simulink library "UltraStick120_Aero_Lib"  (Simulink 8.0)
settings: Solver=ode45  StartTime=0.0  StopTime=10.0  RelTol=1e-3
values from neighbouring files (symbols this model uses):
  AC = miniMUTT_config    [UAV_config.m]    (also in UAV_modelconfig.mat = )
libraries: simulink x2
settings Model: Creator=austinmurch  LastModifiedBy=brtaylor

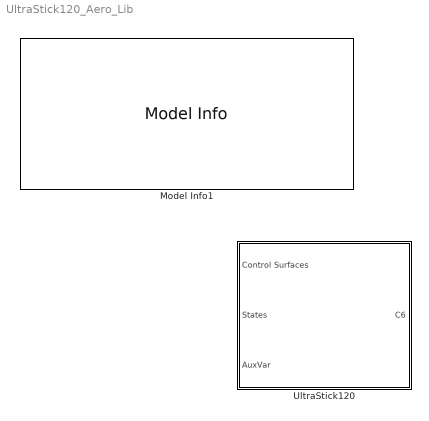
== system UltraStick120_Aero_Lib ==
  Model Info1 : simulink/Model-Wide Utilities/Model Info  InitialBlockCM=None  BlockCM=None  Frame=on  DisplayStringWithTags=|  HorizontalTextAlignment=Left  LeftAlignmentValue=0.02  SourceBlockDiagram=UltraStick120_Aero_Lib  TagMaxNumber=20
      | MODEL INFORMATION
      | FASER Aerodynamic Model Library
      | 
      | University of Minnesota
      | Aerospace Engineering and Mechanics
      | Copyright 2011 Regents of the University of Minnesota. All rights reserved.
      | 
      | == SVN Info ==
      | Last modified by %<LastModifiedBy> on %<LastModificationDate>
  UltraStick120 : Subsystem

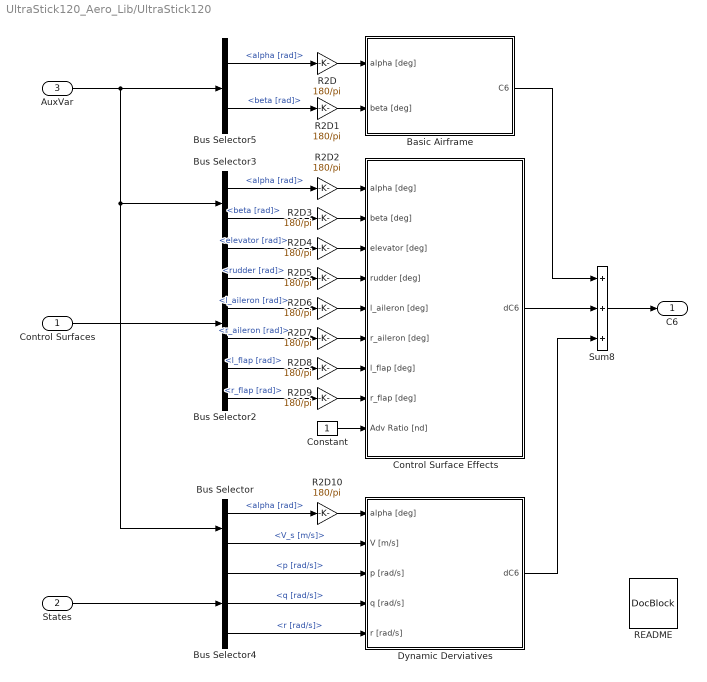
== system UltraStick120_Aero_Lib/UltraStick120 ==
  Control Surfaces : Inport
  States : Inport  Port=2
  AuxVar : Inport  Port=3
  Basic Airframe : Subsystem
  Bus Selector : BusSelector  OutputSignals=WindAxesParam.alpha [rad],WindAxesParam.V_s [m/s]
  Bus Selector2 : BusSelector  OutputSignals=elevator [rad],rudder [rad],l_aileron [rad],r_aileron [rad],l_flap [rad],r_flap [rad]
  Bus Selector3 : BusSelector  OutputSignals=WindAxesParam.alpha [rad],WindAxesParam.beta [rad]
  Bus Selector4 : BusSelector  OutputSignals=AngVel [rad/s].p [rad/s],AngVel [rad/s].q [rad/s],AngVel [rad/s].r [rad/s]
  Bus Selector5 : BusSelector  OutputSignals=WindAxesParam.alpha [rad],WindAxesParam.beta [rad]
  Constant : Constant
  Control Surface Effects : Subsystem
  Dynamic Derviatives : Subsystem
  R2D{,1..10} (11 alike) : Gain  Gain=180/pi
  README : simulink/Model-Wide Utilities/DocBlock  DocumentType=Text
  Sum8 : Sum  Inputs=+++  SaturateOnIntegerOverflow=on  InputSameDT=on  OutDataTypeStr=Inherit: Same as first input
  C6 : Outport
  wires:
  R2D10/1 -> Dynamic Derviatives/1(alpha [deg])
  Bus Selector4/3 -> Dynamic Derviatives/5(r [rad/s])  "<r [rad/s]>"
  Bus Selector4/2 -> Dynamic Derviatives/4(q [rad/s])  "<q [rad/s]>"
  Bus Selector4/1 -> Dynamic Derviatives/3(p [rad/s])  "<p [rad/s]>"
  Bus Selector3/2 -> R2D3/1  "<beta [rad]>"
  Bus Selector3/1 -> R2D2/1  "<alpha [rad]>"
  Bus Selector2/1 -> R2D4/1  "<elevator [rad]>"
  Control Surfaces/1 -> Bus Selector2/1
  Constant/1 -> Control Surface Effects/9(Adv Ratio [nd])
  Basic Airframe/1(C6) -> Sum8/1
  Control Surface Effects/1(dC6) -> Sum8/2
  Dynamic Derviatives/1(dC6) -> Sum8/3
  Sum8/1 -> C6/1
  R2D/1 -> Basic Airframe/1(alpha [deg])
  R2D1/1 -> Basic Airframe/2(beta [deg])
  R2D2/1 -> Control Surface Effects/1(alpha [deg])
  R2D3/1 -> Control Surface Effects/2(beta [deg])
  R2D4/1 -> Control Surface Effects/3(elevator [deg])
  Bus Selector2/2 -> R2D5/1  "<rudder [rad]>"
  R2D5/1 -> Control Surface Effects/4(rudder [deg])
  Bus Selector2/3 -> R2D6/1  "<l_aileron [rad]>"
  Bus Selector2/4 -> R2D7/1  "<r_aileron [rad]>"
  Bus Selector2/5 -> R2D8/1  "<l_flap [rad]>"
  Bus Selector2/6 -> R2D9/1  "<r_flap [rad]>"
  R2D6/1 -> Control Surface Effects/5(l_aileron [deg])
  R2D7/1 -> Control Surface Effects/6(r_aileron [deg])
  R2D8/1 -> Control Surface Effects/7(l_flap [deg])
  R2D9/1 -> Control Surface Effects/8(r_flap [deg])
  Bus Selector5/2 -> R2D1/1  "<beta [rad]>"
  Bus Selector5/1 -> R2D/1  "<alpha [rad]>"
  AuxVar/1 -> Bus Selector/1, Bus Selector3/1, Bus Selector5/1
  Bus Selector/1 -> R2D10/1  "<alpha [rad]>"
  Bus Selector/2 -> Dynamic Derviatives/2(V [m/s])  "<V_s [m/s]>"
  States/1 -> Bus Selector4/1

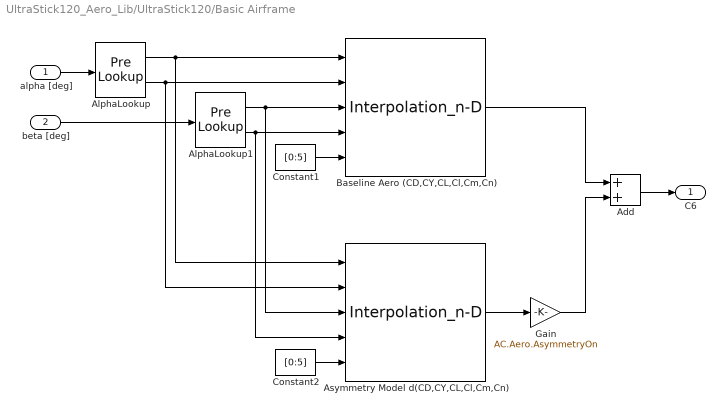
== system UltraStick120_Aero_Lib/UltraStick120/Basic Airframe ==
  alpha [deg] : Inport
  beta [deg] : Inport  Port=2
  Add : Sum
  AlphaLookup : PreLookup  BreakpointsData=AC.Aero.C6_bas.alpha  IndexSearchMethod=Linear search  BeginIndexSearchUsingPreviousIndexResult=on  ExtrapMethod=Linear
  AlphaLookup1 : PreLookup  BreakpointsData=AC.Aero.C6_bas.beta  IndexSearchMethod=Linear search  BeginIndexSearchUsingPreviousIndexResult=on  ExtrapMethod=Linear
  Asymmetry Model d(CD,CY,CL,Cl,Cm,Cn) : Interpolation_n-D  NumberOfTableDimensions=3  Table=AC.Aero.dC6_asym.data  NumSelectionDims=1
      settings: InputPortMap=u0,u1,u2,u3,u4
  Baseline Aero (CD,CY,CL,Cl,Cm,Cn) : Interpolation_n-D  NumberOfTableDimensions=3  Table=AC.Aero.C6_bas.data  NumSelectionDims=1
      settings: InputPortMap=u0,u1,u2,u3,u4
  Constant1 : Constant  Value=[0:5]  OutDataTypeStr=uint32
  Constant2 : Constant  Value=[0:5]  OutDataTypeStr=uint32
  Gain : Gain  Gain=AC.Aero.AsymmetryOn
  C6 : Outport
  wires:
  alpha [deg]/1 -> AlphaLookup/1
  beta [deg]/1 -> AlphaLookup1/1
  AlphaLookup/1 -> Baseline Aero (CD,CY,CL,Cl,Cm,Cn)/1, Asymmetry Model d(CD,CY,CL,Cl,Cm,Cn)/1
  AlphaLookup/2 -> Baseline Aero (CD,CY,CL,Cl,Cm,Cn)/2, Asymmetry Model d(CD,CY,CL,Cl,Cm,Cn)/2
  AlphaLookup1/1 -> Baseline Aero (CD,CY,CL,Cl,Cm,Cn)/3, Asymmetry Model d(CD,CY,CL,Cl,Cm,Cn)/3
  AlphaLookup1/2 -> Baseline Aero (CD,CY,CL,Cl,Cm,Cn)/4, Asymmetry Model d(CD,CY,CL,Cl,Cm,Cn)/4
  Constant1/1 -> Baseline Aero (CD,CY,CL,Cl,Cm,Cn)/5
  Constant2/1 -> Asymmetry Model d(CD,CY,CL,Cl,Cm,Cn)/5
  Baseline Aero (CD,CY,CL,Cl,Cm,Cn)/1 -> Add/1
  Asymmetry Model d(CD,CY,CL,Cl,Cm,Cn)/1 -> Gain/1
  Add/1 -> C6/1
  Gain/1 -> Add/2

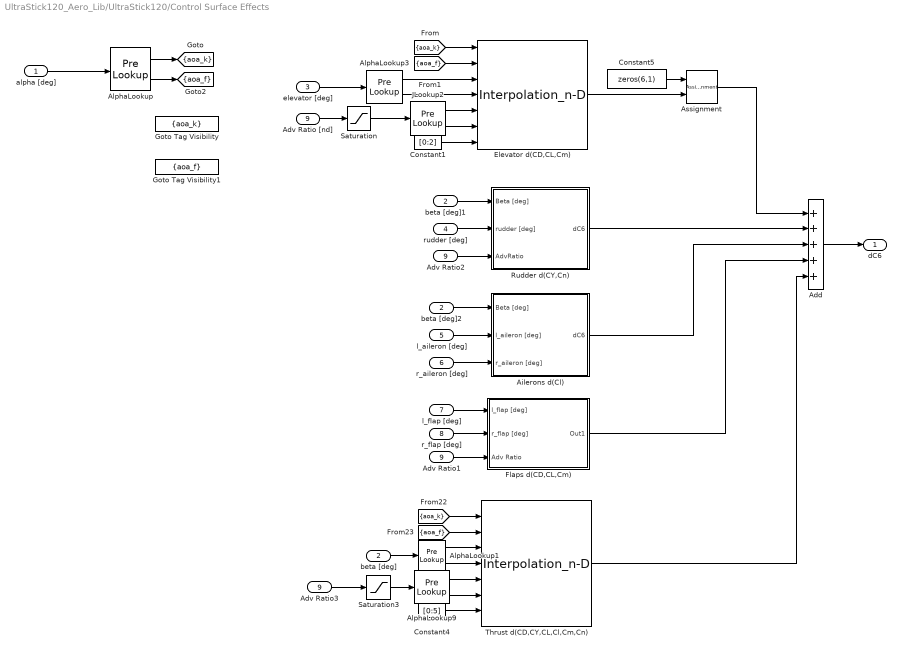
== system UltraStick120_Aero_Lib/UltraStick120/Control Surface Effects ==
  alpha [deg] : Inport
  beta [deg] : Inport  Port=2  PortDimensions=1
  elevator [deg] : Inport  Port=3  PortDimensions=1
  rudder [deg] : Inport  Port=4  PortDimensions=1
  l_aileron [deg] : Inport  Port=5  PortDimensions=1
  r_aileron [deg] : Inport  Port=6  PortDimensions=1
  l_flap [deg] : Inport  Port=7  PortDimensions=1
  r_flap [deg] : Inport  Port=8  PortDimensions=1
  Adv Ratio [nd] : Inport  Port=9
  Add : Sum  Inputs=+++++
  Adv Ratio1 : InportShadow  Port=9
  Adv Ratio2 : InportShadow  Port=9
  Adv Ratio3 : InportShadow  Port=9
  Ailerons d(Cl) : Subsystem
  AlphaLookup : PreLookup  BreakpointsData=AC.Aero.C6_bas.alpha  IndexSearchMethod=Linear search  BeginIndexSearchUsingPreviousIndexResult=on  ExtrapMethod=Linear  UseLastBreakpoint=on
  AlphaLookup1 : PreLookup  BreakpointsData=AC.Aero.C6_bas.beta  IndexSearchMethod=Linear search  BeginIndexSearchUsingPreviousIndexResult=on  ExtrapMethod=Linear  UseLastBreakpoint=on
  AlphaLookup3 : PreLookup  BreakpointsData=AC.Aero.dC3_ele.ele  IndexSearchMethod=Linear search  BeginIndexSearchUsingPreviousIndexResult=on  ExtrapMethod=Linear  UseLastBreakpoint=on
  AlphaLookup9 : PreLookup  BreakpointsData=AC.Aero.dC6_pow.J  IndexSearchMethod=Linear search  BeginIndexSearchUsingPreviousIndexResult=on  ExtrapMethod=Linear  UseLastBreakpoint=on
  Assignment : Assignment  IndexOptions=Index vector (dialog)  Indices=[1 3 5]  OutputSizes=[1 1]
  Constant1 : Constant  Value=[0:2]  OutDataTypeStr=uint32
  Constant4 : Constant  Value=[0:5]  OutDataTypeStr=uint32
  Constant5 : Constant  Value=zeros(6,1)
  Elevator d(CD,CL,Cm) : Interpolation_n-D  NumberOfTableDimensions=4  Table=AC.Aero.dC3_ele.data  NumSelectionDims=1
      settings: InputPortMap=u0,u1,u2,u3,u4,u5,u6
  Flaps d(CD,CL,Cm) : Subsystem
  Goto Tag Visibility : GotoTagVisibility  GotoTag=aoa_k
  Goto Tag Visibility1 : GotoTagVisibility  GotoTag=aoa_f
  JLookup2 : PreLookup  BreakpointsData=AC.Aero.dC3_ele.J  IndexSearchMethod=Linear search  BeginIndexSearchUsingPreviousIndexResult=on  ExtrapMethod=Linear  UseLastBreakpoint=on
  Rudder d(CY,Cn) : Subsystem
  Saturation : Saturate  UpperLimit=max(AC.Aero.dC3_ele.J)  LowerLimit=min(AC.Aero.dC3_ele.J)
  Saturation3 : Saturate  UpperLimit=max(AC.Aero.dC6_pow.J)+eps  LowerLimit=min(AC.Aero.dC6_pow.J)+eps
  Thrust d(CD,CY,CL,Cl,Cm,Cn) : Interpolation_n-D  NumberOfTableDimensions=4  Table=AC.Aero.dC6_pow.data  NumSelectionDims=1
      settings: InputPortMap=u0,u1,u2,u3,u4,u5,u6
  beta [deg]1 : InportShadow  Port=2  PortDimensions=1
  beta [deg]2 : InportShadow  Port=2  PortDimensions=1
  dC6 : Outport  PortDimensions=6
  tag scope: aoa_f=scoped, aoa_k=scoped
  wires:
  alpha [deg]/1 -> AlphaLookup/1
  beta [deg]/1 -> AlphaLookup1/1
  AlphaLookup/1 -> [aoa_k]
  AlphaLookup/2 -> [aoa_f]
  Constant1/1 -> Elevator d(CD,CL,Cm)/7
  [aoa_k] -> Elevator d(CD,CL,Cm)/1
  [aoa_f] -> Elevator d(CD,CL,Cm)/2
  elevator [deg]/1 -> AlphaLookup3/1
  AlphaLookup3/1 -> Elevator d(CD,CL,Cm)/3
  AlphaLookup3/2 -> Elevator d(CD,CL,Cm)/4
  [aoa_k] -> Thrust d(CD,CY,CL,Cl,Cm,Cn)/1
  [aoa_f] -> Thrust d(CD,CY,CL,Cl,Cm,Cn)/2
  AlphaLookup1/1 -> Thrust d(CD,CY,CL,Cl,Cm,Cn)/3
  AlphaLookup1/2 -> Thrust d(CD,CY,CL,Cl,Cm,Cn)/4
  Constant4/1 -> Thrust d(CD,CY,CL,Cl,Cm,Cn)/7
  Elevator d(CD,CL,Cm)/1 -> Assignment/2
  Constant5/1 -> Assignment/1
  Assignment/1 -> Add/1
  Add/1 -> dC6/1
  JLookup2/1 -> Elevator d(CD,CL,Cm)/5
  JLookup2/2 -> Elevator d(CD,CL,Cm)/6
  AlphaLookup9/1 -> Thrust d(CD,CY,CL,Cl,Cm,Cn)/5
  AlphaLookup9/2 -> Thrust d(CD,CY,CL,Cl,Cm,Cn)/6
  Adv Ratio3/1 -> Saturation3/1
  Adv Ratio [nd]/1 -> Saturation/1
  Saturation/1 -> JLookup2/1
  Saturation3/1 -> AlphaLookup9/1
  beta [deg]1/1 -> Rudder d(CY,Cn)/1(Beta [deg])
  rudder [deg]/1 -> Rudder d(CY,Cn)/2(rudder [deg])
  Adv Ratio2/1 -> Rudder d(CY,Cn)/3(AdvRatio)
  r_aileron [deg]/1 -> Ailerons d(Cl)/3(r_aileron [deg])
  l_aileron [deg]/1 -> Ailerons d(Cl)/2(l_aileron [deg])
  beta [deg]2/1 -> Ailerons d(Cl)/1(Beta [deg])
  Adv Ratio1/1 -> Flaps d(CD,CL,Cm)/3(Adv Ratio)
  r_flap [deg]/1 -> Flaps d(CD,CL,Cm)/2(r_flap [deg])
  l_flap [deg]/1 -> Flaps d(CD,CL,Cm)/1(l_flap [deg])
  Rudder d(CY,Cn)/1(dC6) -> Add/2
  Ailerons d(Cl)/1(dC6) -> Add/3
  Flaps d(CD,CL,Cm)/1(Out1) -> Add/4
  Thrust d(CD,CY,CL,Cl,Cm,Cn)/1 -> Add/5

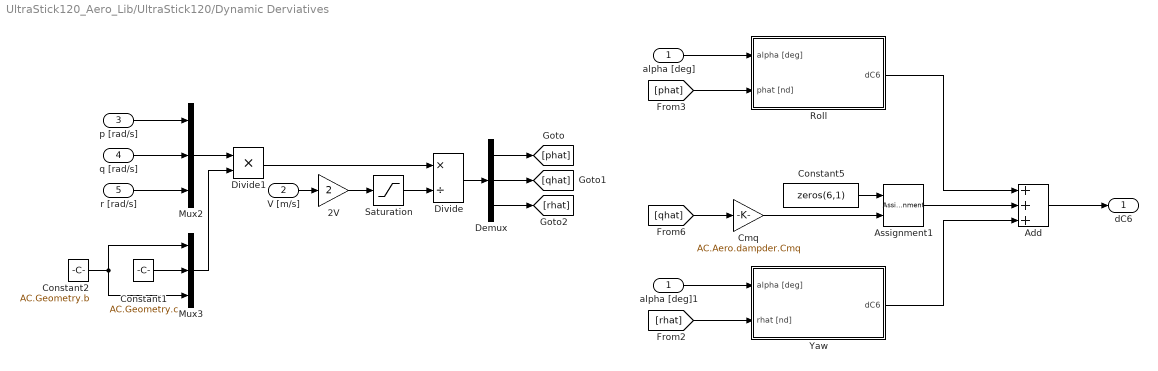
== system UltraStick120_Aero_Lib/UltraStick120/Dynamic Derviatives ==
  alpha [deg] : Inport
  V [m/s] : Inport  Port=2
  p [rad/s] : Inport  Port=3
  q [rad/s] : Inport  Port=4
  r [rad/s] : Inport  Port=5
  2V : Gain  Gain=2
  Add : Sum  Inputs=+++
  Assignment1 : Assignment  IndexOptions=Index vector (dialog)  Indices=5  OutputSizes=[1 1]
  Cmq : Gain  Gain=AC.Aero.dampder.Cmq
  Constant1 : Constant  Value=AC.Geometry.c
  Constant2 : Constant  Value=AC.Geometry.b
  Constant5 : Constant  Value=zeros(6,1)
  Demux : Demux  Outputs=3
  Divide : Product  Inputs=*/
  Divide1 : Product  Inputs=**
  Mux2 : Mux  Inputs=3
  Mux3 : Mux  Inputs=3
  Roll : Subsystem
  Saturation : Saturate  UpperLimit=Inf  LowerLimit=0.001
  Yaw : Subsystem
  alpha [deg]1 : InportShadow
  dC6 : Outport
  wires:
  Yaw/1(dC6) -> Add/3
  Assignment1/1 -> Add/2
  Roll/1(dC6) -> Add/1
  alpha [deg]1/1 -> Yaw/1(alpha [deg])
  alpha [deg]/1 -> Roll/1(alpha [deg])
  Constant5/1 -> Assignment1/1
  [rhat] -> Yaw/2(rhat [nd])
  [phat] -> Roll/2(phat [nd])
  Cmq/1 -> Assignment1/2
  [qhat] -> Cmq/1
  Add/1 -> dC6/1
  V [m/s]/1 -> 2V/1
  2V/1 -> Saturation/1
  Saturation/1 -> Divide/2
  Divide/1 -> Demux/1
  Demux/1 -> [phat]
  Demux/2 -> [qhat]
  Demux/3 -> [rhat]
  Mux2/1 -> Divide1/1
  Divide1/1 -> Divide/1
  Mux3/1 -> Divide1/2
  p [rad/s]/1 -> Mux2/1
  q [rad/s]/1 -> Mux2/2
  r [rad/s]/1 -> Mux2/3
  Constant1/1 -> Mux3/2
  Constant2/1 -> Mux3/1, Mux3/3

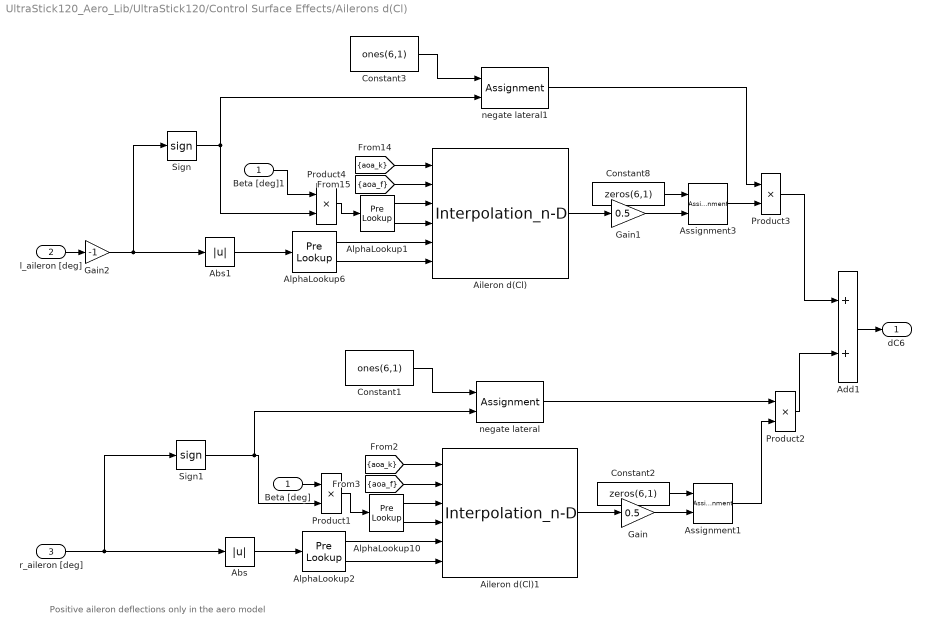
== system UltraStick120_Aero_Lib/UltraStick120/Control Surface Effects/Ailerons d(Cl) ==
  note: Positive aileron deflections only in the aero model
  Beta [deg] : Inport  PortDimensions=1
  l_aileron [deg] : Inport  Port=2  PortDimensions=1
  r_aileron [deg] : Inport  Port=3  PortDimensions=1
  Abs : Abs
  Abs1 : Abs
  Add1 : Sum
  Aileron d(Cl) : Interpolation_n-D  NumberOfTableDimensions=3  Table=AC.Aero.dC1_ail.data
      settings: InputPortMap=u0,u1,u2,u3,u4,u5
  Aileron d(Cl)1 : Interpolation_n-D  NumberOfTableDimensions=3  Table=AC.Aero.dC1_ail.data
      settings: InputPortMap=u0,u1,u2,u3,u4,u5
  AlphaLookup1 : PreLookup  BreakpointsData=AC.Aero.dC1_ail.beta  IndexSearchMethod=Linear search  BeginIndexSearchUsingPreviousIndexResult=on  ExtrapMethod=Linear  UseLastBreakpoint=on
  AlphaLookup10 : PreLookup  BreakpointsData=AC.Aero.dC1_ail.beta  IndexSearchMethod=Linear search  BeginIndexSearchUsingPreviousIndexResult=on  ExtrapMethod=Linear  UseLastBreakpoint=on
  AlphaLookup2 : PreLookup  BreakpointsData=AC.Aero.dC1_ail.ail  IndexSearchMethod=Linear search  BeginIndexSearchUsingPreviousIndexResult=on  ExtrapMethod=Linear
  AlphaLookup6 : PreLookup  BreakpointsData=AC.Aero.dC1_ail.ail  IndexSearchMethod=Linear search  BeginIndexSearchUsingPreviousIndexResult=on  ExtrapMethod=Linear
  Assignment1 : Assignment  IndexOptions=Index vector (dialog)  Indices=4  OutputSizes=[1 1]
  Assignment3 : Assignment  IndexOptions=Index vector (dialog)  Indices=4  OutputSizes=[1 1]
  Beta [deg]1 : InportShadow  PortDimensions=1
  Constant1 : Constant  Value=ones(6,1)
  Constant2 : Constant  Value=zeros(6,1)
  Constant3 : Constant  Value=ones(6,1)
  Constant8 : Constant  Value=zeros(6,1)
  Gain : Gain  Gain=0.5
  Gain1 : Gain  Gain=0.5
  Gain2 : Gain  Gain=-1
  Product{1..4} (4 alike) : Product  RndMeth=Zero
  Sign : Signum
  Sign1 : Signum
  negate lateral : Assignment  IndexMode=Zero-based  IndexOptions=Index vector (dialog)  Indices=[1 3 5]  OutputSizes=[1 1]
  negate lateral1 : Assignment  IndexMode=Zero-based  IndexOptions=Index vector (dialog)  Indices=[1 3 5]  OutputSizes=[1 1]
  dC6 : Outport
  wires:
  [aoa_k] -> Aileron d(Cl)/1
  [aoa_f] -> Aileron d(Cl)/2
  AlphaLookup1/2 -> Aileron d(Cl)/4
  AlphaLookup6/1 -> Aileron d(Cl)/5
  AlphaLookup6/2 -> Aileron d(Cl)/6
  Aileron d(Cl)/1 -> Gain1/1
  Constant8/1 -> Assignment3/1
  [aoa_k] -> Aileron d(Cl)1/1
  [aoa_f] -> Aileron d(Cl)1/2
  AlphaLookup2/1 -> Aileron d(Cl)1/5
  AlphaLookup2/2 -> Aileron d(Cl)1/6
  r_aileron [deg]/1 -> Abs/1, Sign1/1
  l_aileron [deg]/1 -> Gain2/1
  Add1/1 -> dC6/1
  Abs/1 -> AlphaLookup2/1
  AlphaLookup10/1 -> Aileron d(Cl)1/3
  AlphaLookup10/2 -> Aileron d(Cl)1/4
  Product1/1 -> AlphaLookup10/1
  Sign1/1 -> Product1/2, negate lateral/2
  Beta [deg]/1 -> Product1/1
  Constant1/1 -> negate lateral/1
  Constant2/1 -> Assignment1/1
  Aileron d(Cl)1/1 -> Gain/1
  Assignment1/1 -> Product2/2
  negate lateral/1 -> Product2/1
  Product2/1 -> Add1/2
  Assignment3/1 -> Product3/2
  Product3/1 -> Add1/1
  Constant3/1 -> negate lateral1/1
  negate lateral1/1 -> Product3/1
  Abs1/1 -> AlphaLookup6/1
  AlphaLookup1/1 -> Aileron d(Cl)/3
  Product4/1 -> AlphaLookup1/1
  Sign/1 -> Product4/2, negate lateral1/2
  Beta [deg]1/1 -> Product4/1
  Gain2/1 -> Abs1/1, Sign/1
  Gain/1 -> Assignment1/2
  Gain1/1 -> Assignment3/2

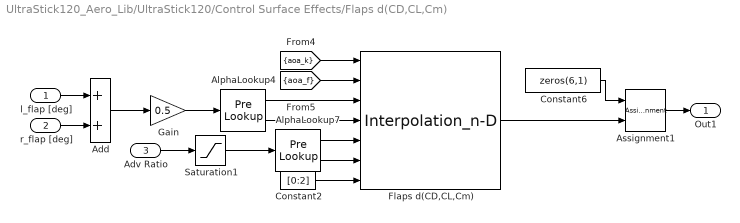
== system UltraStick120_Aero_Lib/UltraStick120/Control Surface Effects/Flaps d(CD,CL,Cm) ==
  l_flap [deg] : Inport  PortDimensions=1
  r_flap [deg] : Inport  Port=2  PortDimensions=1
  Adv Ratio : Inport  Port=3
  Add : Sum
  AlphaLookup4 : PreLookup  BreakpointsData=AC.Aero.dC3_flap.flap  IndexSearchMethod=Linear search  BeginIndexSearchUsingPreviousIndexResult=on  ExtrapMethod=Linear
  AlphaLookup7 : PreLookup  BreakpointsData=AC.Aero.dC3_flap.J  IndexSearchMethod=Linear search  BeginIndexSearchUsingPreviousIndexResult=on  ExtrapMethod=Linear  UseLastBreakpoint=on
  Assignment1 : Assignment  IndexOptions=Index vector (dialog)  Indices=[1 3 5]  OutputSizes=[1 1]
  Constant2 : Constant  Value=[0:2]  OutDataTypeStr=uint32
  Constant6 : Constant  Value=zeros(6,1)
  Flaps d(CD,CL,Cm) : Interpolation_n-D  NumberOfTableDimensions=4  Table=AC.Aero.dC3_flap.data  NumSelectionDims=1
      settings: InputPortMap=u0,u1,u2,u3,u4,u5,u6
  Gain : Gain  Gain=0.5
  Saturation1 : Saturate  UpperLimit=max(AC.Aero.dC3_flap.J)  LowerLimit=min(AC.Aero.dC3_flap.J)
  Out1 : Outport
  wires:
  Constant2/1 -> Flaps d(CD,CL,Cm)/7
  [aoa_k] -> Flaps d(CD,CL,Cm)/1
  [aoa_f] -> Flaps d(CD,CL,Cm)/2
  AlphaLookup4/1 -> Flaps d(CD,CL,Cm)/3
  AlphaLookup4/2 -> Flaps d(CD,CL,Cm)/4
  Flaps d(CD,CL,Cm)/1 -> Assignment1/2
  Constant6/1 -> Assignment1/1
  AlphaLookup7/1 -> Flaps d(CD,CL,Cm)/5
  AlphaLookup7/2 -> Flaps d(CD,CL,Cm)/6
  Adv Ratio/1 -> Saturation1/1
  Saturation1/1 -> AlphaLookup7/1
  Assignment1/1 -> Out1/1
  l_flap [deg]/1 -> Add/1
  r_flap [deg]/1 -> Add/2
  Add/1 -> Gain/1
  Gain/1 -> AlphaLookup4/1

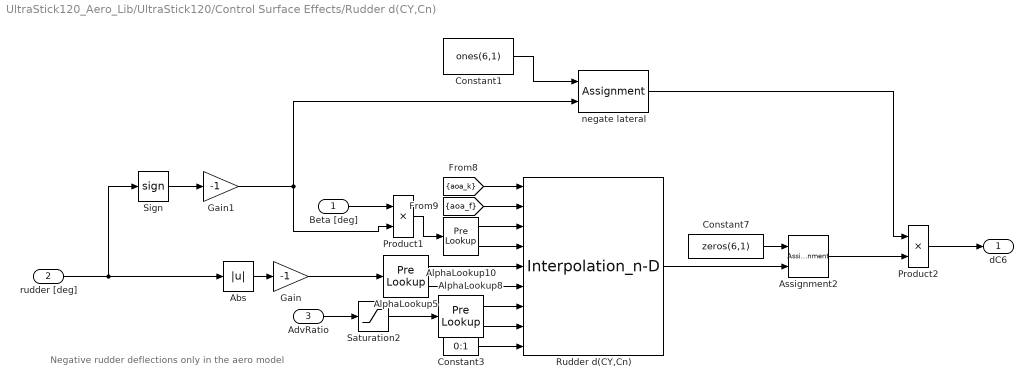
== system UltraStick120_Aero_Lib/UltraStick120/Control Surface Effects/Rudder d(CY,Cn) ==
  note: Negative rudder deflections only in the aero model
  Beta [deg] : Inport  PortDimensions=1
  rudder [deg] : Inport  Port=2  PortDimensions=1
  AdvRatio : Inport  Port=3
  Abs : Abs
  AlphaLookup10 : PreLookup  BreakpointsData=AC.Aero.dC2_rud.beta  IndexSearchMethod=Linear search  BeginIndexSearchUsingPreviousIndexResult=on  ExtrapMethod=Linear  UseLastBreakpoint=on
  AlphaLookup5 : PreLookup  BreakpointsData=AC.Aero.dC2_rud.rud  IndexSearchMethod=Linear search  BeginIndexSearchUsingPreviousIndexResult=on  ExtrapMethod=Linear
  AlphaLookup8 : PreLookup  BreakpointsData=AC.Aero.dC2_rud.J  IndexSearchMethod=Linear search  BeginIndexSearchUsingPreviousIndexResult=on  ExtrapMethod=Linear  UseLastBreakpoint=on
  Assignment2 : Assignment  IndexOptions=Index vector (dialog)  Indices=[2 6]  OutputSizes=[1 1]
  Constant1 : Constant  Value=ones(6,1)
  Constant3 : Constant  Value=0:1  OutDataTypeStr=uint32
  Constant7 : Constant  Value=zeros(6,1)
  Gain : Gain  Gain=-1
  Gain1 : Gain  Gain=-1
  Product1 : Product  RndMeth=Zero
  Product2 : Product  RndMeth=Zero
  Rudder d(CY,Cn) : Interpolation_n-D  NumberOfTableDimensions=5  Table=AC.Aero.dC2_rud.data  NumSelectionDims=1
      settings: InputPortMap=u0,u1,u2,u3,u4,u5,u6,u7,u8
  Saturation2 : Saturate  UpperLimit=max(AC.Aero.dC2_rud.J)  LowerLimit=min(AC.Aero.dC2_rud.J)
  Sign : Signum
  negate lateral : Assignment  IndexMode=Zero-based  IndexOptions=Index vector (dialog)  Indices=[1 3 5]  OutputSizes=[1 1]
  dC6 : Outport
  wires:
  [aoa_k] -> Rudder d(CY,Cn)/1
  [aoa_f] -> Rudder d(CY,Cn)/2
  Constant3/1 -> Rudder d(CY,Cn)/9
  AlphaLookup5/1 -> Rudder d(CY,Cn)/5
  AlphaLookup5/2 -> Rudder d(CY,Cn)/6
  Rudder d(CY,Cn)/1 -> Assignment2/2
  Constant7/1 -> Assignment2/1
  AlphaLookup8/1 -> Rudder d(CY,Cn)/7
  AlphaLookup8/2 -> Rudder d(CY,Cn)/8
  AdvRatio/1 -> Saturation2/1
  Saturation2/1 -> AlphaLookup8/1
  AlphaLookup10/1 -> Rudder d(CY,Cn)/3
  AlphaLookup10/2 -> Rudder d(CY,Cn)/4
  Abs/1 -> Gain/1
  rudder [deg]/1 -> Abs/1, Sign/1
  Gain/1 -> AlphaLookup5/1
  Beta [deg]/1 -> Product1/1
  Product1/1 -> AlphaLookup10/1
  Sign/1 -> Gain1/1
  Constant1/1 -> negate lateral/1
  Product2/1 -> dC6/1
  Assignment2/1 -> Product2/2
  negate lateral/1 -> Product2/1
  Gain1/1 -> Product1/2, negate lateral/2

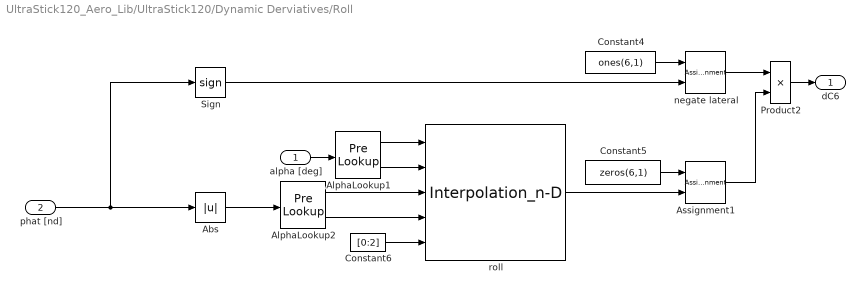
== system UltraStick120_Aero_Lib/UltraStick120/Dynamic Derviatives/Roll ==
  alpha [deg] : Inport
  phat [nd] : Inport  Port=2
  Abs : Abs
  AlphaLookup1 : PreLookup  BreakpointsData=AC.Aero.dC3_p.alpha  IndexSearchMethod=Linear search  BeginIndexSearchUsingPreviousIndexResult=on  ExtrapMethod=Linear
  AlphaLookup2 : PreLookup  BreakpointsData=AC.Aero.dC3_p.phat  IndexSearchMethod=Linear search  BeginIndexSearchUsingPreviousIndexResult=on  ExtrapMethod=Linear
  Assignment1 : Assignment  IndexOptions=Index vector (dialog)  Indices=[2 4 6]  OutputSizes=[1 1]
  Constant4 : Constant  Value=ones(6,1)
  Constant5 : Constant  Value=zeros(6,1)
  Constant6 : Constant  Value=[0:2]  OutDataTypeStr=uint32
  Product2 : Product  RndMeth=Zero
  Sign : Signum
  negate lateral : Assignment  IndexOptions=Index vector (dialog)  Indices=[2 4 6]  OutputSizes=[1 1]
  roll : Interpolation_n-D  NumberOfTableDimensions=3  Table=AC.Aero.dC3_p.data  NumSelectionDims=1
      settings: InputPortMap=u0,u1,u2,u3,u4
  dC6 : Outport
  wires:
  alpha [deg]/1 -> AlphaLookup1/1
  Product2/1 -> dC6/1
  AlphaLookup1/2 -> roll/2
  AlphaLookup1/1 -> roll/1
  Constant6/1 -> roll/5
  AlphaLookup2/2 -> roll/4
  AlphaLookup2/1 -> roll/3
  phat [nd]/1 -> Abs/1, Sign/1
  Abs/1 -> AlphaLookup2/1
  Constant4/1 -> negate lateral/1
  Constant5/1 -> Assignment1/1
  roll/1 -> Assignment1/2
  Assignment1/1 -> Product2/2
  negate lateral/1 -> Product2/1
  Sign/1 -> negate lateral/2

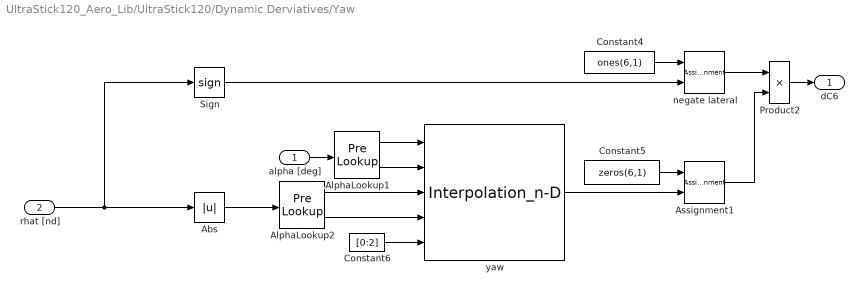
== system UltraStick120_Aero_Lib/UltraStick120/Dynamic Derviatives/Yaw ==
  alpha [deg] : Inport
  rhat [nd] : Inport  Port=2
  Abs : Abs
  AlphaLookup1 : PreLookup  BreakpointsData=AC.Aero.dC3_r.alpha  IndexSearchMethod=Linear search  BeginIndexSearchUsingPreviousIndexResult=on  ExtrapMethod=Linear
  AlphaLookup2 : PreLookup  BreakpointsData=AC.Aero.dC3_r.rhat  IndexSearchMethod=Linear search  BeginIndexSearchUsingPreviousIndexResult=on  ExtrapMethod=Linear
  Assignment1 : Assignment  IndexOptions=Index vector (dialog)  Indices=[2 4 6]  OutputSizes=[1 1]
  Constant4 : Constant  Value=ones(6,1)
  Constant5 : Constant  Value=zeros(6,1)
  Constant6 : Constant  Value=[0:2]  OutDataTypeStr=uint32
  Product2 : Product  RndMeth=Zero
  Sign : Signum
  negate lateral : Assignment  IndexOptions=Index vector (dialog)  Indices=[2 4 6]  OutputSizes=[1 1]
  yaw : Interpolation_n-D  NumberOfTableDimensions=3  Table=AC.Aero.dC3_r.data  NumSelectionDims=1
      settings: InputPortMap=u0,u1,u2,u3,u4
  dC6 : Outport
  wires:
  Assignment1/1 -> Product2/2
  yaw/1 -> Assignment1/2
  Constant5/1 -> Assignment1/1
  Abs/1 -> AlphaLookup2/1
  rhat [nd]/1 -> Abs/1, Sign/1
  AlphaLookup2/1 -> yaw/3
  AlphaLookup2/2 -> yaw/4
  Constant6/1 -> yaw/5
  AlphaLookup1/1 -> yaw/1
  AlphaLookup1/2 -> yaw/2
  Product2/1 -> dC6/1
  alpha [deg]/1 -> AlphaLookup1/1
  Constant4/1 -> negate lateral/1
  negate lateral/1 -> Product2/1
  Sign/1 -> negate lateral/2
